simulink model "vtol_roll"  (R2020b)
settings: Solver=VariableStepAuto  StartTime=0.0  StopTime=10  RelTol=1e-3
values from neighbouring files (symbols this model uses):
  d_threshold = 1    [VTOL_pitch_Simulink_constants.m]    (also in VTOL_roll_Simulink_constants.m; VTOL_yaw_Simulink_constants.m)
  Fmax = 10    [VTOL_pitch_Simulink_constants.m]    (also in VTOL_roll_Simulink_constants.m = 71220)
  Jxx = Iyy + Izz    [VTOL_roll_Simulink_constants.m]
  l = 3.68    [VTOL_roll_Simulink_constants.m]    (also in VTOL_yaw_Simulink_constants.m)
  n_threshold = 1    [VTOL_pitch_Simulink_constants.m]    (also in VTOL_roll_Simulink_constants.m; VTOL_yaw_Simulink_constants.m)
  tau = 10    [VTOL_pitch_Simulink_constants.m]    (also in VTOL_roll_Simulink_constants.m = 5)
  threshold = -1    [VTOL_pitch_Simulink_constants.m]
  V_wind = 1    [VTOL_pitch_Simulink_constants.m]
libraries: simulink x1, aerolibwind2 x1, pid_lib x1
settings Model: Creator=Tomo  LastModifiedBy=Tomo

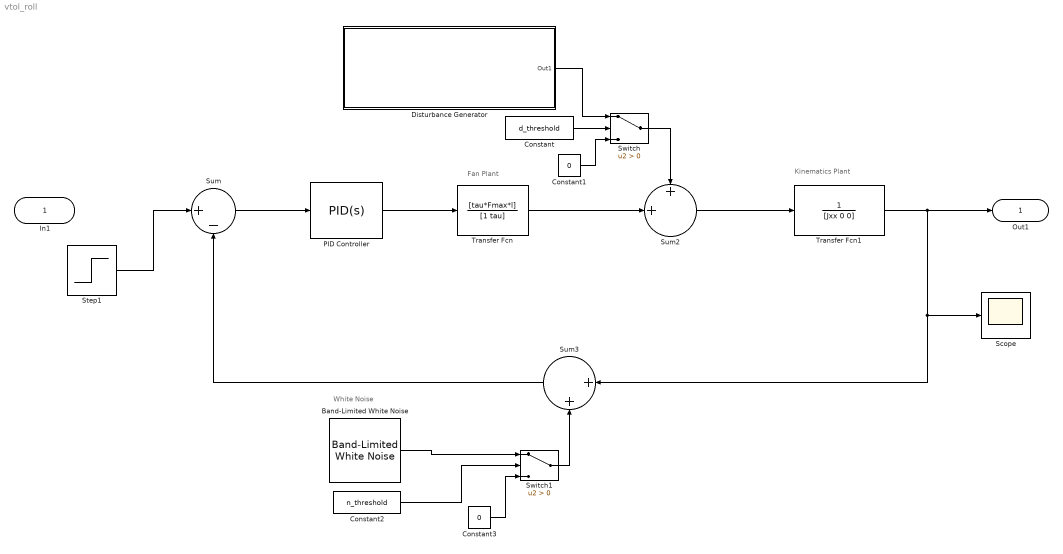
== system vtol_roll ==
  note: Kinematics Plant
  note: Fan Plant
  note: White Noise
  In1 : Inport
  Band-Limited White Noise : simulink/Sources/Band-Limited White Noise  Cov=[0.01]  Ts=0.01  seed=[23341]
  Constant : Constant  Value=d_threshold
  Constant1 : Constant  Value=0
  Constant2 : Constant  Value=n_threshold
  Constant3 : Constant  Value=0
  Disturbance Generator : Subsystem
  PID Controller : pid_lib/PID Controller  Controller=PID  Form=Parallel  TimeDomain=Continuous-time  UseExternalTs=off  SampleTime=-1  IntegratorMethod=Forward Euler  FilterMethod=Forward Euler  ControllerParametersSource=internal  P=1.81481547825078e-05  I=1.81171194402346e-12  D=0.3129809309805  UseFilter=on  N=23.7738638769895  TunerSelectOption=Transfer Function Based (PID Tuner App)  InitialConditionSource=internal  InitialConditionForIntegrator=0  InitialConditionForFilter=0  DifferentiatorICPrevScaledInput=0  ExternalReset=none  TrackingMode=off  Kt=1  LimitOutput=off  SatLimitsSource=internal  UpperSaturationLimit=inf  LowerSaturationLimit=-inf  LinearizeAsGain=on  AntiWindupMode=none  Kb=1  POutMin=[]  POutMax=[]  IOutMin=[]  IOutMax=[]  DOutMin=[]  DOutMax=[]  NOutMin=[]  NOutMax=[]  SumOutMin=[]  SumOutMax=[]  SaturationOutMin=[]  SaturationOutMax=[]  PParamMin=[]  PParamMax=[]  IParamMin=[]  IParamMax=[]  DParamMin=[]  DParamMax=[]  NParamMin=[]  NParamMax=[]  KbParamMin=[]  KbParamMax=[]  KtParamMin=[]  KtParamMax=[]  KbOutMin=[]  KbOutMax=[]  KtOutMin=[]  KtOutMax=[]  IntegratorOutMin=[]  IntegratorOutMax=[]  FilterOutMin=[]  FilterOutMax=[]  SumI1OutMin=[]  SumI1OutMax=[]  SumI2OutMin=[]  SumI2OutMax=[]  SumI3OutMin=[]  SumI3OutMax=[]  SumI4OutMin=[]  SumI4OutMax=[]  SumDOutMin=[]  SumDOutMax=[]  DifferentiatorOutMin=[]  DifferentiatorOutMax=[]  FilterDiffOutCoefMin=[]  FilterDiffOutCoefMax=[]  ReciprocalOutMin=[]  ReciprocalOutMax=[]  SumDenOutMin=[]  SumDenOutMax=[]  SumNumOutMin=[]  SumNumOutMax=[]  DivideOutMin=[]  DivideOutMax=[]  UdiffTsProdOutMin=[]  UdiffTsProdOutMax=[]  NTsProdOutMin=[]  NTsProdOutMax=[]  UintegralTsProdOutMin=[]  UintegralTsProdOutMax=[]  UngainTsProdOutMin=[]  UngainTsProdOutMax=[]  IntegratorContinuousStateAttributes=''  IntegratorStateMustResolveToSignalObject=off  IntegratorRTWStateStorageClass=Auto  FilterContinuousStateAttributes=''  FilterStateMustResolveToSignalObject=off  FilterRTWStateStorageClass=Auto  ParallelPVariant=InternalParameters  IdealPVariant=Disabled  IVariant=InternalParameters  DVariant=InternalParameters  IntegratorVariant=Continuous  SatVariant=Disabled  AWVariant=Passthrough  PCopyVariant=Disabled  TRVariant=Disabled  FdbkBlocksVariant=Forward  IdealPFdbkVariant=Disabled  SatFdbkVariant=Disabled  DerivativeFilterVariant=ContFilter  NVariant=InternalParameters  NCopyVariant=Disabled  FilterICVariant=InternalICsFilter  IntegratorICVariant=InternalICs  ExternalResetVariant=Disabled  TRSumVariant=Passthrough  SumFdbkVariant=Disabled  SumVariant=Sum_PID  TsampFilterVariant=InternalTs  TsampNgainVariant=Passthrough  TsampIntegralVariant=Passthrough  ExternalSaturationOutDataTypeStr=Inherit: Same as second input
  Scope : Scope
  Step1 : Step  SampleTime=0
  Sum : Sum  Inputs=|+-
  Sum2 : Sum  Inputs=++|
  Sum3 : Sum  Inputs=|++
  Switch : Switch  Criteria=u2 > Threshold
  Switch1 : Switch  Criteria=u2 > Threshold
  Transfer Fcn : TransferFcn  Numerator=[tau*Fmax*l]  Denominator=[1 tau]
  Transfer Fcn1 : TransferFcn  Denominator=[Jxx 0 0]
  Out1 : Outport
  wires:
  Sum/1 -> PID Controller/1
  PID Controller/1 -> Transfer Fcn/1
  Transfer Fcn1/1 -> Sum3/1, Scope/1, Out1/1
  Step1/1 -> Sum/1
  Transfer Fcn/1 -> Sum2/2
  Sum2/1 -> Transfer Fcn1/1
  Disturbance Generator/1(Out1) -> Switch/1
  Constant/1 -> Switch/2
  Constant1/1 -> Switch/3
  Sum3/1 -> Sum/2
  Switch/1 -> Sum2/1
  Band-Limited White Noise/1 -> Switch1/1
  Constant2/1 -> Switch1/2
  Constant3/1 -> Switch1/3
  Switch1/1 -> Sum3/2

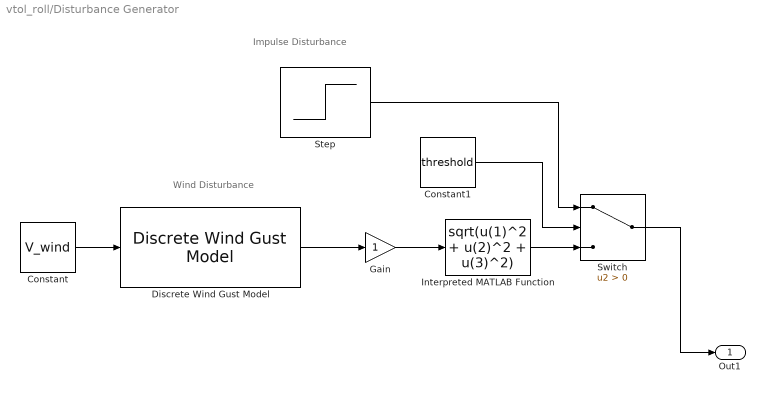
== system vtol_roll/Disturbance Generator ==
  note: Wind Disturbance
  note: Impulse Disturbance
  Constant : Constant  Value=V_wind
  Constant1 : Constant  Value=threshold
  Discrete Wind Gust Model : aerolibwind2/Discrete Wind Gust Model  units=Metric (MKS)  Gx=off  Gy=on  Gz=off  t_0=5  d_m=[120 120 80]  v_m=[3.5 3.5 3.0]
  Gain : Gain
  Interpreted MATLAB Function : MATLABFcn  MATLABFcn=sqrt(u(1)^2 + u(2)^2 + u(3)^2)
  Step : Step  SampleTime=0
  Switch : Switch  Criteria=u2 > Threshold
  Out1 : Outport
  wires:
  Switch/1 -> Out1/1
  Constant/1 -> Discrete Wind Gust Model/1
  Interpreted MATLAB Function/1 -> Switch/3
  Constant1/1 -> Switch/2
  Step/1 -> Switch/1
  Discrete Wind Gust Model/1 -> Gain/1
  Gain/1 -> Interpreted MATLAB Function/1
